simulink model "synchro_v2"  (R2020b)
settings: Solver=FixedStepAuto  StartTime=0.0  StopTime=2  FixedStep=Ts  RelTol=1e-3
values from neighbouring files (symbols this model uses):
  m = 5/100    (= 0.05)    [synchro_parameters_v1.m]
  Sbase = 1    [synchro_parameters_v1.m]
  Ts = 1/Fs    (= 0.0001)    [synchro_parameters_v1.m]
  Vbase = 1    [synchro_parameters_v1.m]
  w_droop = 10*2*pi    (= 62.8318530718)    [synchro_parameters_v1.m]
  w_pll = 10*2*pi    (= 62.8318530718)    [synchro_parameters_v1.m]
  w_tau = 1e3*2*pi    (= 6283.18530718)    [synchro_parameters_v1.m]
  Wbase = 2*pi*50    (= 314.159265359)    [synchro_parameters_v1.m]
undefined symbols (not defined in the file or in its folder): DiscIntNeverNeededParam
libraries: powerlib x36, SimplexPS x34, Simplex_PowerSystems x4
(part 1 of 2)
settings Model: Creator=admin_user  LastModifiedBy=admin_user

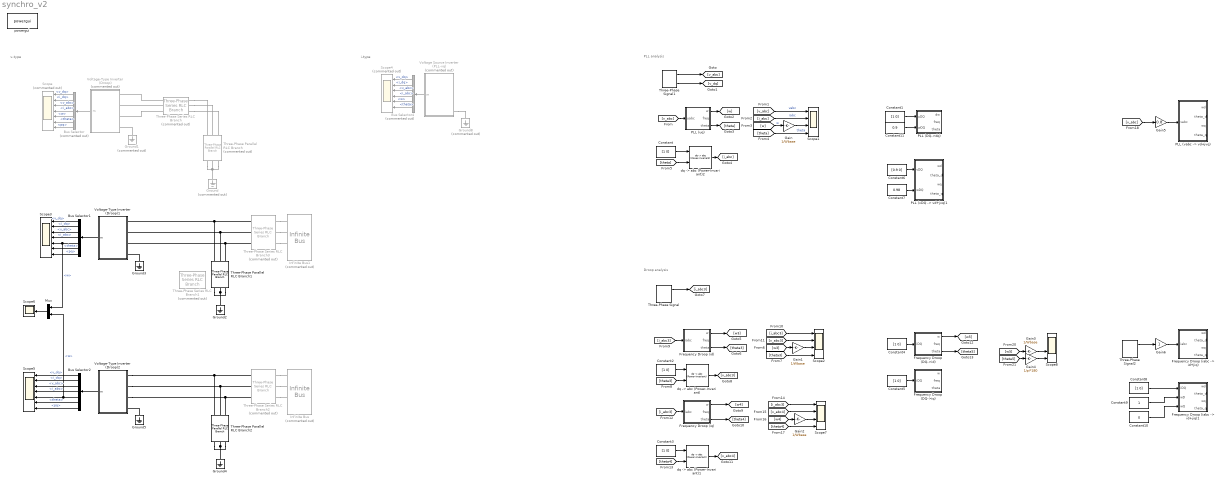
== system synchro_v2 ==
  note: Droop analysis
  note: PLL analysis
  note: i-type
  note: v-type
  Bus Selector : BusSelector  Commented=on  OutputSignals=v_dq,i_dq,v_abc,i_abc,w,theta,pq
  Bus Selector1 : BusSelector  OutputSignals=v_dq,i_dq,v_abc,i_abc,w,theta,pq
  Bus Selector2 : BusSelector  OutputSignals=v_dq,i_dq,v_abc,i_abc,w,theta,pq
  Bus Selector4 : BusSelector  Commented=on  OutputSignals=v_dq,i_dq,v_abc,i_abc,w,theta
  Constant{,1..5,8} (7 alike) : Constant  Value=[1 0]
  Constant10 : Constant  Value=0
  Constant11 : Constant  Value=0.9
  Constant6 : Constant  Value=[0.9 0]
  Constant7 : Constant  Value=0.98
  Constant9 : Constant
  "Frequency Droop (iabc -> id+jiq)" : Subsystem  AncestorBlock=|  mask{Ts=Ts, Sbase=Sbase, Vbase=Vbase, Wbase=Wbase, m=m, w_tau=w_droop, theta_d0=0, theta_q0=0, id0=0, iq0=0, wd0=1, wq0=0}
      | SimplexPS/Frequency Droop
      | (iabc -> id+jiq)
      mask prompts: Ts "Ts (s), sampling period"; Sbase "Sbase (VA), base power"; Vbase "Vbase (V), base voltage"; Wbase "Wbase (s), base frequency"; m "m (pu), droop gain"; w_tau "w_tau (pu), low-pass filter bandwidth"; theta_d0 "theta_d0 (rad/s), initial d-axis angle"; theta_q0 "theta_q0 (rad/s), initial q-axis angle"; id0 "id0 (pu), d-axis current setting point"; iq0 "iq0 (pu), q-axis current setting point"; wd0 "wd0 (pu), d-axis angular frequency setting point"; wq0 "wq0 (pu), q-axis angular frequency setting point"
  "Frequency Droop (iabc -> id+jiq)1" : Subsystem  AncestorBlock=|  mask{Ts=Ts, Sbase=Sbase, Vbase=Vbase, Wbase=Wbase, m=m, w_tau=w_droop, theta_d0=0, theta_q0=0, id0=0, iq0=0, wd0=1, wq0=0}
      | SimplexPS/Frequency Droop
      | (iabc -> id+jiq)1
      mask prompts: Ts "Ts (s), sampling period"; Sbase "Sbase (VA), base power"; Vbase "Vbase (V), base voltage"; Wbase "Wbase (s), base frequency"; m "m (pu), droop gain"; w_tau "w_tau (pu), low-pass filter bandwidth"; theta_d0 "theta_d0 (rad/s), initial d-axis angle"; theta_q0 "theta_q0 (rad/s), initial q-axis angle"; id0 "id0 (pu), d-axis current setting point"; iq0 "iq0 (pu), q-axis current setting point"; wd0 "wd0 (pu), d-axis angular frequency setting point"; wq0 "wq0 (pu), q-axis angular frequency setting point"
  Frequency Droop (DQ->id) : Subsystem  AncestorBlock=SimplexPS/Frequency Droop (id)  mask{Ts=Ts, Sbase=Sbase, Vbase=Vbase, Wbase=Wbase, m=m, w_tau=w_droop, theta0=0, P0=0, W0=1}
      mask prompts: Ts "Ts (s), samping period"; Sbase "Sbase (VA), base power"; Vbase "Vbase (V), base voltage"; Wbase "Wbase (rad/s), base angular frequency"; m "m (pu), droop gain"; w_tau "w_tau (rad/s), low-pass filter bandwidth"; theta0 "theta0 (rad), initial angle"; P0 "P0 (pu), power setting point"; W0 "W0 (pu), frequency setting point"
  Frequency Droop (DQ->iq) : Subsystem  AncestorBlock=SimplexPS/Frequency Droop (id)  mask{Ts=Ts, Sbase=Sbase, Vbase=Vbase, Wbase=Wbase, m=m, w_tau=w_droop, theta0=0, P0=0, W0=1}
      mask prompts: Ts "Ts (s), samping period"; Sbase "Sbase (VA), base power"; Vbase "Vbase (V), base voltage"; Wbase "Wbase (rad/s), base angular frequency"; m "m (pu), droop gain"; w_tau "w_tau (rad/s), low-pass filter bandwidth"; theta0 "theta0 (rad), initial angle"; P0 "P0 (pu), power setting point"; W0 "W0 (pu), frequency setting point"
  Frequency Droop (id) : Subsystem  AncestorBlock=SimplexPS/Frequency Droop (id)  mask{Ts=Ts, Sbase=Sbase, Vbase=Vbase, Wbase=Wbase, m=m, w_tau=w_droop, theta0=0, P0=0, W0=1}
      mask prompts: Ts "Ts (s), samping period"; Sbase "Sbase (VA), base power"; Vbase "Vbase (V), base voltage"; Wbase "Wbase (rad/s), base angular frequency"; m "m (pu), droop gain"; w_tau "w_tau (rad/s), low-pass filter bandwidth"; theta0 "theta0 (rad), initial angle"; P0 "P0 (pu), power setting point"; W0 "W0 (pu), frequency setting point"
  Frequency Droop (iq) : Subsystem  AncestorBlock=SimplexPS/Frequency Droop (iq)  mask{Ts=Ts, Sbase=Sbase, Vbase=Vbase, Wbase=Wbase, m=m, w_tau=w_droop, theta0=0, P0=0, W0=1}
      mask prompts: Ts "Ts (s), samping period"; Sbase "Sbase (VA), base power"; Vbase "Vbase (V), base voltage"; Wbase "Wbase (rad/s), base angular frequency"; m "m (pu), droop gain"; w_tau "w_tau (rad/s), low-pass filter bandwidth"; theta0 "theta0 (rad), initial angle"; P0 "P0 (pu), power setting point"; W0 "W0 (pu), frequency setting point"
  Gain{,1..3} (4 alike) : Gain  Gain=1/Wbase
  Gain4 : Gain  Gain=1/pi*180
  Gain5 : Gain  Gain=0.8
  Gain6 : Gain
  Ground : powerlib/Elements/Ground  Commented=on  LConnTagsString=a
  Ground1 : powerlib/Elements/Ground  Commented=on  LConnTagsString=a
  Ground{2..5} (4 alike) : powerlib/Elements/Ground  LConnTagsString=a
  Ground8 : powerlib/Elements/Ground  Commented=on  LConnTagsString=a
  Infinite Bus : SimplexPS/Infinite Bus  Commented=on  Ts=Ts  Sbase=Sbase  Vbase=Vbase  Wbase=Wbase  vd=1  vq=0  theta0=0  w=Wbase  R=1e-30
      settings: SourceProductName=Simplex Power Systems
  Infinite Bus1 : SimplexPS/Infinite Bus  Commented=on  Ts=Ts  Sbase=Sbase  Vbase=Vbase  Wbase=Wbase  vd=1  vq=0  theta0=0  w=Wbase  R=1e-30
      settings: SourceProductName=Simplex Power Systems
  Mux : Mux  Inputs=2
  "PLL (vDQ -> vd+jvq)1" : Subsystem  AncestorBlock=|  mask{Ts=Ts, Wbase=Wbase, Vbase=Vbase, w_pll=w_pll, w_tau=w_tau, theta_d0=pi/4, theta_q0=0}
      | SimplexPS/PLL
      | (vabc -> vd+jvq)
      mask prompts: Ts "Ts (s), sampling period"; Wbase "Wbase (rad/s), frequency base"; Vbase "Vbase (rad/s), voltage base"; w_pll "w_pll (rad/s), PLL bandwidth"; w_tau "w_tau (rad/s), PLL filter"; theta_d0 "theta_d0 (rad), initial d-axis angle"; theta_q0 "theta_q0 (rad), initial q-axis angle"
  "PLL (vabc -> vd+jvq)" : Subsystem  AncestorBlock=|  mask{Ts=Ts, Wbase=Wbase, Vbase=Vbase, w_pll=w_pll, w_tau=w_tau, theta_d0=pi/4, theta_q0=0}
      | SimplexPS/PLL
      | (vabc -> vd+jvq)
      mask prompts: Ts "Ts (s), sampling period"; Wbase "Wbase (rad/s), frequency base"; Vbase "Vbase (rad/s), voltage base"; w_pll "w_pll (rad/s), PLL bandwidth"; w_tau "w_tau (rad/s), PLL filter"; theta_d0 "theta_d0 (rad), initial d-axis angle"; theta_q0 "theta_q0 (rad), initial q-axis angle"
  PLL (DQ->dq) : Subsystem  AncestorBlock=SimplexPS/PLL (uq)  mask{Ts=Ts, Ubase=Vbase, Wbase=Wbase, w_pll=w_pll, w_tau=w_tau, theta0=0}
      mask prompts: Ts "Ts (s), sampling period"; Ubase "Ubase, input base, e.g., Vbase (V), Ibase (A), etc"; Wbase "Wbase (rad/s), frequency base"; w_pll "w_pll (rad/s), PLL bandwidth"; w_tau "w_tau (rad/s), low-pass filter bandwidth"; theta0 "theta0 (rad), initial angle"
  PLL (uq) : Subsystem  AncestorBlock=SimplexPS/PLL (uq)  mask{Ts=Ts, Ubase=Vbase, Wbase=Wbase, w_pll=w_pll, w_tau=w_tau, theta0=0}
      mask prompts: Ts "Ts (s), sampling period"; Ubase "Ubase, input base, e.g., Vbase (V), Ibase (A), etc"; Wbase "Wbase (rad/s), frequency base"; w_pll "w_pll (rad/s), PLL bandwidth"; w_tau "w_tau (rad/s), low-pass filter bandwidth"; theta0 "theta0 (rad), initial angle"
  Scope : Scope  Commented=on  NumInputPorts=7
  Scope{1..2,7..8} (4 alike) : Scope  NumInputPorts=4
  Scope3 : Scope  NumInputPorts=7
  Scope4 : Scope  Commented=on  NumInputPorts=6
  Scope5 : Scope  NumInputPorts=7
  Scope6 : Scope
  Three-Phase Parallel RLC Branch : powerlib/Elements/Three-Phase Parallel RLC Branch  Commented=on  LConnTagsString=A|B|C  RConnTagsString=A|B|C  BranchType=R  Resistance=1  Inductance=1e-3  Capacitance=1e-6  Measurements=None
      settings: SourceProductBaseCode=PS
  Three-Phase Parallel RLC Branch1 : powerlib/Elements/Three-Phase Parallel RLC Branch  LConnTagsString=A|B|C  RConnTagsString=A|B|C  BranchType=R  Resistance=1  Inductance=1e-3  Capacitance=1e-6  Measurements=None
      settings: SourceProductBaseCode=PS
  Three-Phase Parallel RLC Branch2 : powerlib/Elements/Three-Phase Parallel RLC Branch  LConnTagsString=A|B|C  RConnTagsString=A|B|C  BranchType=R  Resistance=1  Inductance=1e-3  Capacitance=1e-6  Measurements=None
      settings: SourceProductBaseCode=PS
  Three-Phase Series RLC Branch{,1..3} (4 alike) : powerlib/Elements/Three-Phase Series RLC Branch  Commented=on  LConnTagsString=A|B|C  RConnTagsString=A|B|C  BranchType=RL  Resistance=0.01  Inductance=0.2/(2*pi*50)  Capacitance=1e-6  Measurements=None
  Three-Phase Signal : SimplexPS/Three-Phase Signal  ud=1  uq=0  w=Wbase*1  theta0=0
      settings: SourceProductName=Simplex Power Systems
  Three-Phase Signal1 : SimplexPS/Three-Phase Signal  ud=1  uq=0  w=Wbase*0.95  theta0=0
      settings: SourceProductName=Simplex Power Systems
  Three-Phase Signal2 : SimplexPS/Three-Phase Signal  ud=1  uq=0  w=Wbase*0.98  theta0=0
      settings: SourceProductName=Simplex Power Systems
  Voltage Source Inverter (PLL-vq) : Subsystem  Commented=on  mask{Sbase=Sbase, Vbase=Vbase, Wbase=Wbase, Ts=Ts, i_d_r=1, i_q_r=0, w_pll=w_pll, w_tau=w_tau}
      mask prompts: Sbase "Sbase (VA), power base"; Vbase "Vbase (V), voltage base"; Wbase "Wbase (rad/s), frequency base"; Ts "Ts (s), samping period"; i_d_r "i_d_r (pu), d-axis current reference"; i_q_r "i_q_r (pu), q-axis current reference"; w_pll "w_pll (rad/s), PLL bandwidth"; w_tau "w_tau (rad/s), PLL filter"
  Voltage-Type Inverter (Droop) : Subsystem  Commented=on  mask{Sbase=Sbase, Vbase=Vbase, Wbase=Wbase, Ts=Ts, v_d0=1, v_q0=0, w0=1, m=m, n=0, P0=0, Q0=0, w_droop=w_droop}
      mask prompts: Sbase "Sbase (VA)"; Vbase "Vbase (V)"; Wbase "Wbase (rad/s)"; Ts "Ts (s)"; v_d0 "v_d0 (pu), d-axis voltage setting point"; v_q0 "v_q0 (pu), q-axis voltage setting point"; w0 "w0 (pu), frequency setting point"; m "m (pu), frequency droop gain"; n "n (pu), voltage droop gain"; P0 "P0 (pu), active power setting point"; Q0 "Q0 (pu), reactive power setting point"; w_droop "w_droop (rad/s), droop bandwidth"
  Voltage-Type Inverter (Droop)1 : Subsystem  mask{Sbase=Sbase, Vbase=Vbase, Wbase=Wbase, Ts=Ts, v_d0=1, v_q0=0, w0=1, m=m, n=0, P0=0, Q0=0, w_droop=w_droop}
      mask prompts: Sbase "Sbase (VA)"; Vbase "Vbase (V)"; Wbase "Wbase (rad/s)"; Ts "Ts (s)"; v_d0 "v_d0 (pu), d-axis voltage setting point"; v_q0 "v_q0 (pu), q-axis voltage setting point"; w0 "w0 (pu), frequency setting point"; m "m (pu), frequency droop gain"; n "n (pu), voltage droop gain"; P0 "P0 (pu), active power setting point"; Q0 "Q0 (pu), reactive power setting point"; w_droop "w_droop (rad/s), droop bandwidth"
  Voltage-Type Inverter (Droop)2 : Subsystem  mask{Sbase=Sbase, Vbase=Vbase, Wbase=Wbase, Ts=Ts, v_d0=1, v_q0=0, w0=1, m=m, n=0, P0=0, Q0=0, w_droop=w_droop}
      mask prompts: Sbase "Sbase (VA)"; Vbase "Vbase (V)"; Wbase "Wbase (rad/s)"; Ts "Ts (s)"; v_d0 "v_d0 (pu), d-axis voltage setting point"; v_q0 "v_q0 (pu), q-axis voltage setting point"; w0 "w0 (pu), frequency setting point"; m "m (pu), frequency droop gain"; n "n (pu), voltage droop gain"; P0 "P0 (pu), active power setting point"; Q0 "Q0 (pu), reactive power setting point"; w_droop "w_droop (rad/s), droop bandwidth"
  "dq -> abc (Power-Invariant)" : SimplexPS/dq -> abc (Power-Invariant)  SystemSampleTime=-1  VariantActivationTime=update diagram  Latency=0  AutoFrameSizeCalculation=off
      settings: SourceProductName=Simplex Power Systems
  "dq -> abc (Power-Invariant)1" : SimplexPS/dq -> abc (Power-Invariant)  SystemSampleTime=-1  VariantActivationTime=update diagram  Latency=0  AutoFrameSizeCalculation=off
      settings: SourceProductName=Simplex Power Systems
  "dq -> abc (Power-Invariant)2" : SimplexPS/dq -> abc (Power-Invariant)  SystemSampleTime=-1  VariantActivationTime=update diagram  Latency=0  AutoFrameSizeCalculation=off
      settings: SourceProductName=Simplex Power Systems
  powergui : powerlib/powergui  Priority=1  SimulationMode=Discrete  SampleTime=Ts  frequency=60  Iterations=50  frequencyindice=0  Pbase=100e6  ErrMax=1e-4  UnitsV=kV  UnitsW=MW  buscounter=0  FunctionMessages=off  echomessages=off  EnableUseOfTLC=off  CurrentSourceSwitches=off  DisableSnubberDevices=off  DisableRonSwitches=off  DisableVfSwitches=off  DisplayEquations=off  AutomaticDiscreteSolvers=off  SolverType=Tustin/Backward Euler (TBE)  Interpol=off  ExternalGateDelay=off  methode=off  Ts=100  x0status=blocks  SPID=on  SwTol=0  HookPort=off  NonlinearTolerance=1e-4  nMaxIteration=100  ContinueOnMaxIteration=off  RestoreLinks=warning  ResistiveCurrentMeasurement=off  Frange=[0:2:500]  Ylog=off  Xlog=on  ShowGrid=off  save=off  variable=ZData  structure=0  ZoomFFT=off  StartTime=0.0  cycles=1  DisplayStyle=1  fundamental=60  FreqAxis=off  MaxFrequency=1000  frequencyindicesteady=1  RmsSteady=1  display=off
  wires:
  Voltage-Type Inverter (Droop)/1(m) -> Bus Selector/1
  Bus Selector/1 -> Scope/1  "<v_dq>"
  Bus Selector/2 -> Scope/2  "<i_dq>"
  Bus Selector/3 -> Scope/3  "<v_abc>"
  Bus Selector/4 -> Scope/4  "<i_abc>"
  Bus Selector/5 -> Scope/5  "<w>"
  Bus Selector/6 -> Scope/6  "<theta>"
  Bus Selector/7 -> Scope/7  "<pq>"
  Bus Selector4/3 -> Scope4/3  "<v_abc>"
  Bus Selector4/4 -> Scope4/4  "<i_abc>"
  Bus Selector4/6 -> Scope4/6  "<theta>"
  Bus Selector4/1 -> Scope4/1  "<v_dq>"
  Voltage Source Inverter (PLL-vq)/1(m) -> Bus Selector4/1
  Bus Selector4/5 -> Scope4/5  "<w>"
  Bus Selector4/2 -> Scope4/2  "<i_dq>"
  [v_abc] -> PLL (uq)/1(uabc)
  [v_abc] -> Scope1/1  "vabc"
  PLL (uq)/3(theta) -> [theta]
  PLL (uq)/1(w) -> [w]
  [theta] -> Scope1/4  "theta"
  Constant/1 -> "dq -> abc (Power-Invariant)2"/1
  [theta] -> "dq -> abc (Power-Invariant)2"/2
  "dq -> abc (Power-Invariant)2"/1 -> [i_abc]
  [i_abc] -> Scope1/2  "iabc"
  Constant1/1 -> PLL (DQ->dq)/1(uDQ)
  Frequency Droop (id)/1(w) -> [w3]
  Frequency Droop (id)/3(theta) -> [theta3]
  [theta3] -> Scope2/4
  Three-Phase Signal/1 -> [i_abc3]
  [i_abc3] -> Frequency Droop (id)/1(iabc)
  Constant2/1 -> "dq -> abc (Power-Invariant)"/1
  [theta3] -> "dq -> abc (Power-Invariant)"/2
  "dq -> abc (Power-Invariant)"/1 -> [v_abc3]
  [i_abc3] -> Scope2/1
  [v_abc3] -> Scope2/2
  Three-Phase Signal1/1 -> [v_abc]
  Three-Phase Signal1/2 -> [v_dq]
  [w] -> Gain/1  "w"
  Gain/1 -> Scope1/3
  [w3] -> Gain1/1
  Gain1/1 -> Scope2/3
  Bus Selector1/5 -> Mux/1, Scope3/5  "<w>"
  Bus Selector1/3 -> Scope3/3  "<v_abc>"
  Bus Selector1/6 -> Scope3/6  "<theta>"
  Bus Selector1/7 -> Scope3/7  "<pq>"
  Bus Selector1/2 -> Scope3/2  "<i_dq>"
  Bus Selector1/4 -> Scope3/4  "<i_abc>"
  Bus Selector1/1 -> Scope3/1  "<v_dq>"
  Voltage-Type Inverter (Droop)1/1(m) -> Bus Selector1/1
  Bus Selector2/2 -> Scope5/2  "<i_dq>"
  Bus Selector2/4 -> Scope5/4  "<i_abc>"
  Bus Selector2/1 -> Scope5/1  "<v_dq>"
  Voltage-Type Inverter (Droop)2/1(m) -> Bus Selector2/1
  Bus Selector2/6 -> Scope5/6  "<theta>"
  Bus Selector2/3 -> Scope5/3  "<v_abc>"
  Bus Selector2/7 -> Scope5/7  "<pq>"
  Bus Selector2/5 -> Mux/2, Scope5/5  "<w>"
  Mux/1 -> Scope6/1
  [i_abc3] -> Frequency Droop (iq)/1(iabc)
  Frequency Droop (iq)/1(w) -> [w4]
  Frequency Droop (iq)/3(theta) -> [theta4]
  [theta4] -> "dq -> abc (Power-Invariant)1"/2
  Constant3/1 -> "dq -> abc (Power-Invariant)1"/1
  "dq -> abc (Power-Invariant)1"/1 -> [v_abc4]
  [theta4] -> Scope7/4
  [w4] -> Gain2/1
  [v_abc4] -> Scope7/2
  [i_abc3] -> Scope7/1
  Gain2/1 -> Scope7/3
  Constant4/1 -> Frequency Droop (DQ->id)/1(iDQ)
  Frequency Droop (DQ->id)/3(theta) -> [theta5]
  Frequency Droop (DQ->id)/1(w) -> [w5]
  Gain3/1 -> Scope8/3
  [w5] -> Gain3/1
  [theta5] -> Gain4/1
  Gain4/1 -> Scope8/4
  Constant5/1 -> Frequency Droop (DQ->iq)/1(iDQ)
  [v_abc] -> Gain5/1
  Gain5/1 -> "PLL (vabc -> vd+jvq)"/1(vabc)
  Gain6/1 -> "Frequency Droop (iabc -> id+jiq)"/1(iabc)
  Constant6/1 -> "PLL (vDQ -> vd+jvq)1"/1(vDQ)
  Constant7/1 -> "PLL (vDQ -> vd+jvq)1"/2(wDQ)
  Three-Phase Signal2/1 -> Gain6/1
  Constant8/1 -> "Frequency Droop (iabc -> id+jiq)1"/1(iDQ)
  Constant9/1 -> "Frequency Droop (iabc -> id+jiq)1"/2(wD)
  Constant10/1 -> "Frequency Droop (iabc -> id+jiq)1"/3(wQ)
  Constant11/1 -> PLL (DQ->dq)/2(wDQ)
  connections:
  Ground/LConn1 -- Three-Phase Parallel RLC Branch/RConn3 -- Three-Phase Parallel RLC Branch/RConn1 -- Three-Phase Parallel RLC Branch/RConn2
  Ground1/LConn1 -- Voltage-Type Inverter (Droop)/LConn4
  Three-Phase Series RLC Branch/RConn1 -- Three-Phase Parallel RLC Branch/LConn1
  Three-Phase Series RLC Branch/RConn2 -- Three-Phase Parallel RLC Branch/LConn2
  Three-Phase Series RLC Branch/RConn3 -- Three-Phase Parallel RLC Branch/LConn3
  Three-Phase Series RLC Branch/LConn1 -- Voltage-Type Inverter (Droop)/LConn1
  Three-Phase Series RLC Branch/LConn2 -- Voltage-Type Inverter (Droop)/LConn2
  Three-Phase Series RLC Branch/LConn3 -- Voltage-Type Inverter (Droop)/LConn3
  Voltage Source Inverter (PLL-vq)/LConn4 -- Ground8/LConn1
  Three-Phase Parallel RLC Branch1/RConn2 -- Ground2/LConn1 -- Three-Phase Parallel RLC Branch1/RConn3 -- Three-Phase Parallel RLC Branch1/RConn1
  Three-Phase Parallel RLC Branch1/LConn3 -- Voltage-Type Inverter (Droop)1/LConn3 -- Three-Phase Series RLC Branch3/LConn3
  Ground3/LConn1 -- Voltage-Type Inverter (Droop)1/LConn4
  Three-Phase Parallel RLC Branch1/LConn2 -- Voltage-Type Inverter (Droop)1/LConn2 -- Three-Phase Series RLC Branch3/LConn2
  Three-Phase Parallel RLC Branch1/LConn1 -- Voltage-Type Inverter (Droop)1/LConn1 -- Three-Phase Series RLC Branch3/LConn1
  Three-Phase Parallel RLC Branch2/RConn2 -- Ground4/LConn1 -- Three-Phase Parallel RLC Branch2/RConn3 -- Three-Phase Parallel RLC Branch2/RConn1
  Voltage-Type Inverter (Droop)2/LConn3 -- Three-Phase Series RLC Branch2/LConn3 -- Three-Phase Parallel RLC Branch2/LConn3
  Ground5/LConn1 -- Voltage-Type Inverter (Droop)2/LConn4
  Voltage-Type Inverter (Droop)2/LConn1 -- Three-Phase Parallel RLC Branch2/LConn1 -- Three-Phase Series RLC Branch2/LConn1
  Voltage-Type Inverter (Droop)2/LConn2 -- Three-Phase Series RLC Branch2/LConn2 -- Three-Phase Parallel RLC Branch2/LConn2
  Three-Phase Series RLC Branch2/RConn1 -- Infinite Bus/LConn1
  Three-Phase Series RLC Branch2/RConn2 -- Infinite Bus/LConn2
  Three-Phase Series RLC Branch2/RConn3 -- Infinite Bus/LConn3
  Three-Phase Series RLC Branch3/RConn1 -- Infinite Bus1/LConn1
  Three-Phase Series RLC Branch3/RConn3 -- Infinite Bus1/LConn3
  Three-Phase Series RLC Branch3/RConn2 -- Infinite Bus1/LConn2

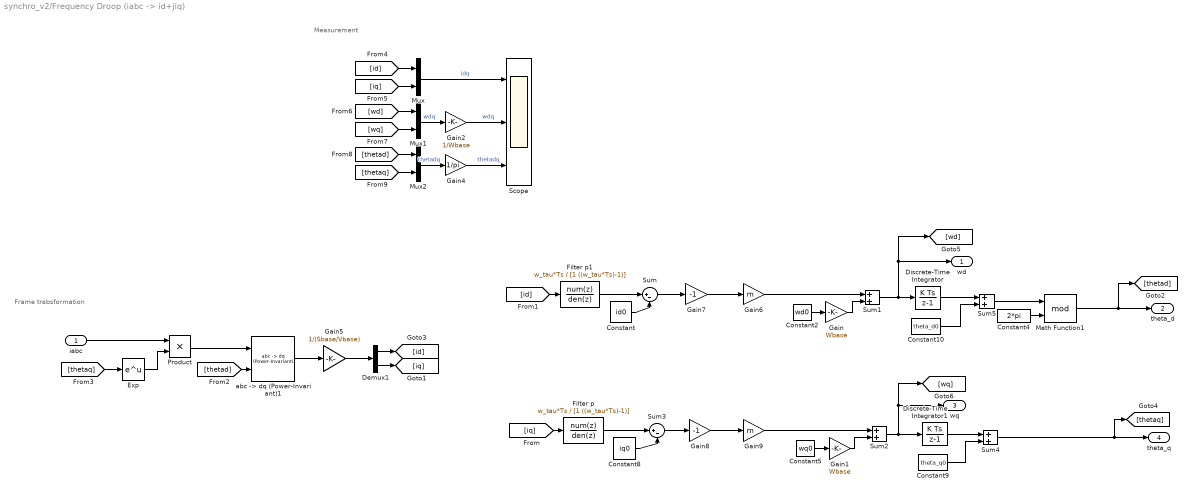
== system synchro_v2/Frequency Droop (iabc -> id+jiq) ==
  note: Frame trabsformation
  note: Measurement
  iabc : Inport
  Constant : Constant  Value=id0
  Constant10 : Constant  Value=theta_d0
  Constant2 : Constant  Value=wd0
  Constant4 : Constant  Value=2*pi
  Constant5 : Constant  Value=wq0
  Constant8 : Constant  Value=iq0
  Constant9 : Constant  Value=theta_q0
  Demux1 : Demux  Outputs=2
  Discrete-Time Integrator : DiscreteIntegrator  SampleTime=Ts  ICPrevOutput=DiscIntNeverNeededParam  ICPrevScaledInput=DiscIntNeverNeededParam
  Discrete-Time Integrator1 : DiscreteIntegrator  SampleTime=Ts  ICPrevOutput=DiscIntNeverNeededParam  ICPrevScaledInput=DiscIntNeverNeededParam
  Exp : Math  SignedPower=on  SaturateOnIntegerOverflow=on
  Filter p : DiscreteTransferFcn  Numerator=w_tau*Ts  Denominator=[1 ((w_tau*Ts)-1)]  SampleTime=Ts
  Filter p1 : DiscreteTransferFcn  Numerator=w_tau*Ts  Denominator=[1 ((w_tau*Ts)-1)]  SampleTime=Ts
  Gain : Gain  Gain=Wbase
  Gain1 : Gain  Gain=Wbase
  Gain2 : Gain  Gain=1/Wbase
  Gain4 : Gain  Gain=1/pi
  Gain5 : Gain  Gain=1/(Sbase/Vbase)
  Gain6 : Gain  Gain=m
  Gain7 : Gain  Gain=-1
  Gain8 : Gain  Gain=-1
  Gain9 : Gain  Gain=m
  Math Function1 : Math  Operator=mod  SignedPower=on  SaturateOnIntegerOverflow=on
  Mux : Mux  Inputs=2
  Mux1 : Mux  Inputs=2
  Mux2 : Mux  Inputs=2
  Product : Product
  Scope : Scope  NumInputPorts=3
  Sum : Sum  Inputs=|+-
  Sum{1..2,4..5} (4 alike) : Sum
  Sum3 : Sum  Inputs=|+-
  "abc -> dq (Power-Invariant)1" : SimplexPS/abc -> dq (Power-Invariant)  SystemSampleTime=-1  VariantActivationTime=update diagram  Latency=0  AutoFrameSizeCalculation=off
      settings: SourceProductName=Simplex Power Systems
  wd : Outport
  theta_d : Outport  Port=2
  wq : Outport  Port=3
  theta_q : Outport  Port=4
  wires:
  Gain8/1 -> Gain9/1
  Sum3/1 -> Gain8/1
  Gain7/1 -> Gain6/1
  Gain6/1 -> Sum1/1
  Gain9/1 -> Sum2/1
  Filter p1/1 -> Sum/1
  [iq] -> Filter p/1
  [wq] -> Mux1/2
  iabc/1 -> Product/1
  [id] -> Filter p1/1
  [thetad] -> "abc -> dq (Power-Invariant)1"/2
  Filter p/1 -> Sum3/1
  Discrete-Time Integrator1/1 -> Sum4/1
  Product/1 -> "abc -> dq (Power-Invariant)1"/1
  [id] -> Mux/1
  Constant10/1 -> Sum5/2
  [thetaq] -> Exp/1
  Gain/1 -> Sum1/2
  Constant5/1 -> Gain1/1
  [thetad] -> Mux2/1
  Exp/1 -> Product/2
  Mux1/1 -> Gain2/1  "wdq"
  [thetaq] -> Mux2/2
  [iq] -> Mux/2
  Constant/1 -> Sum/2
  [wd] -> Mux1/1
  Constant8/1 -> Sum3/2
  Sum5/1 -> Math Function1/1
  Demux1/1 -> [id]
  Sum4/1 -> [thetaq], theta_q/1
  Constant4/1 -> Math Function1/2
  Sum/1 -> Gain7/1
  Demux1/2 -> [iq]
  Gain4/1 -> Scope/3  "thetadq"
  Mux/1 -> Scope/1  "idq"
  Gain5/1 -> Demux1/1
  Constant9/1 -> Sum4/2
  Gain1/1 -> Sum2/2
  Mux2/1 -> Gain4/1  "thetadq"
  Sum1/1 -> Discrete-Time Integrator/1, [wd], wd/1
  Math Function1/1 -> [thetad], theta_d/1
  "abc -> dq (Power-Invariant)1"/1 -> Gain5/1
  Discrete-Time Integrator/1 -> Sum5/1
  Sum2/1 -> [wq], wq/1, Discrete-Time Integrator1/1
  Gain2/1 -> Scope/2  "wdq"
  Constant2/1 -> Gain/1

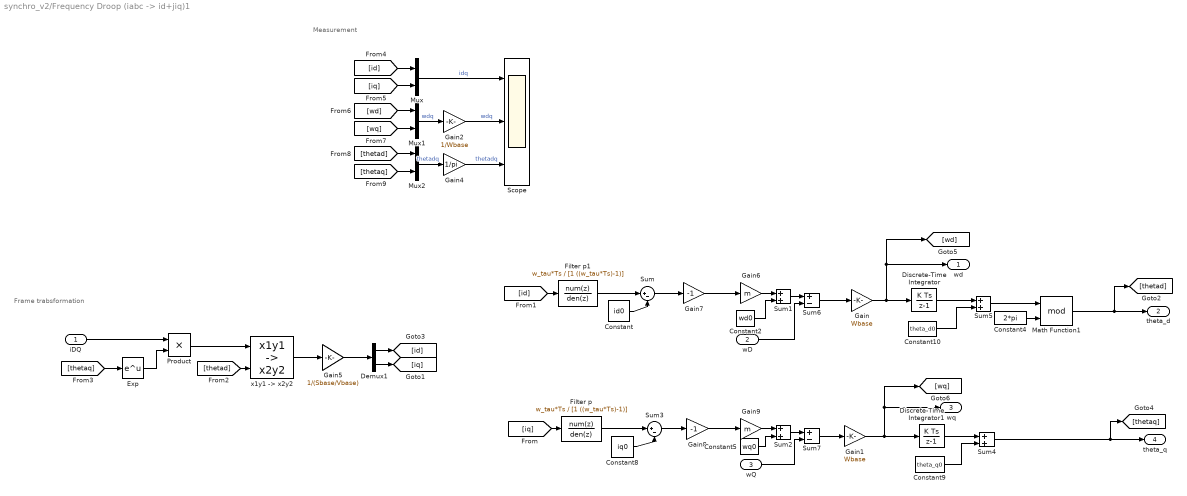
== system synchro_v2/Frequency Droop (iabc -> id+jiq)1 ==
  note: Measurement
  note: Frame trabsformation
  iDQ : Inport
  wD : Inport  Port=2
  wQ : Inport  Port=3
  Constant : Constant  Value=id0
  Constant10 : Constant  Value=theta_d0
  Constant2 : Constant  Value=wd0
  Constant4 : Constant  Value=2*pi
  Constant5 : Constant  Value=wq0
  Constant8 : Constant  Value=iq0
  Constant9 : Constant  Value=theta_q0
  Demux1 : Demux  Outputs=2
  Discrete-Time Integrator : DiscreteIntegrator  SampleTime=Ts  ICPrevOutput=DiscIntNeverNeededParam  ICPrevScaledInput=DiscIntNeverNeededParam
  Discrete-Time Integrator1 : DiscreteIntegrator  SampleTime=Ts  ICPrevOutput=DiscIntNeverNeededParam  ICPrevScaledInput=DiscIntNeverNeededParam
  Exp : Math  SignedPower=on  SaturateOnIntegerOverflow=on
  Filter p : DiscreteTransferFcn  Numerator=w_tau*Ts  Denominator=[1 ((w_tau*Ts)-1)]  SampleTime=Ts
  Filter p1 : DiscreteTransferFcn  Numerator=w_tau*Ts  Denominator=[1 ((w_tau*Ts)-1)]  SampleTime=Ts
  Gain : Gain  Gain=Wbase
  Gain1 : Gain  Gain=Wbase
  Gain2 : Gain  Gain=1/Wbase
  Gain4 : Gain  Gain=1/pi
  Gain5 : Gain  Gain=1/(Sbase/Vbase)
  Gain6 : Gain  Gain=m
  Gain7 : Gain  Gain=-1
  Gain8 : Gain  Gain=-1
  Gain9 : Gain  Gain=m
  Math Function1 : Math  Operator=mod  SignedPower=on  SaturateOnIntegerOverflow=on
  Mux : Mux  Inputs=2
  Mux1 : Mux  Inputs=2
  Mux2 : Mux  Inputs=2
  Product : Product
  Scope : Scope  NumInputPorts=3
  Sum : Sum  Inputs=|+-
  Sum{1..2,4..5} (4 alike) : Sum
  Sum3 : Sum  Inputs=|+-
  Sum6 : Sum  Inputs=+-
  Sum7 : Sum  Inputs=+-
  "x1y1 -> x2y2" : SimplexPS/x1y1 -> x2y2  SystemSampleTime=-1  VariantActivationTime=update diagram  Latency=0  AutoFrameSizeCalculation=off
      settings: SourceProductName=Simplex Power Systems
  wd : Outport
  theta_d : Outport  Port=2
  wq : Outport  Port=3
  theta_q : Outport  Port=4
  wires:
  Gain2/1 -> Scope/2  "wdq"
  Discrete-Time Integrator/1 -> Sum5/1
  "x1y1 -> x2y2"/1 -> Gain5/1
  Math Function1/1 -> theta_d/1, [thetad]
  Mux2/1 -> Gain4/1  "thetadq"
  Constant5/1 -> Sum2/2
  Constant9/1 -> Sum4/2
  Gain5/1 -> Demux1/1
  Mux/1 -> Scope/1  "idq"
  Gain4/1 -> Scope/3  "thetadq"
  Demux1/2 -> [iq]
  Sum/1 -> Gain7/1
  Constant4/1 -> Math Function1/2
  Sum4/1 -> theta_q/1, [thetaq]
  Demux1/1 -> [id]
  Sum5/1 -> Math Function1/1
  Constant8/1 -> Sum3/2
  [wd] -> Mux1/1
  Constant/1 -> Sum/2
  [iq] -> Mux/2
  [thetaq] -> Mux2/2
  Mux1/1 -> Gain2/1  "wdq"
  Exp/1 -> Product/2
  [thetad] -> Mux2/1
  Constant2/1 -> Sum1/2
  [thetaq] -> Exp/1
  Constant10/1 -> Sum5/2
  [id] -> Mux/1
  Product/1 -> "x1y1 -> x2y2"/1
  Discrete-Time Integrator1/1 -> Sum4/1
  Filter p/1 -> Sum3/1
  [thetad] -> "x1y1 -> x2y2"/2
  [id] -> Filter p1/1
  iDQ/1 -> Product/1
  [wq] -> Mux1/2
  [iq] -> Filter p/1
  Filter p1/1 -> Sum/1
  Gain9/1 -> Sum2/1
  Gain6/1 -> Sum1/1
  Gain7/1 -> Gain6/1
  Sum3/1 -> Gain8/1
  Gain8/1 -> Gain9/1
  Gain/1 -> [wd], wd/1, Discrete-Time Integrator/1
  Sum1/1 -> Sum6/1
  Sum6/1 -> Gain/1
  wD/1 -> Sum6/2
  Gain1/1 -> [wq], wq/1, Discrete-Time Integrator1/1
  Sum2/1 -> Sum7/1
  Sum7/1 -> Gain1/1
  wQ/1 -> Sum7/2

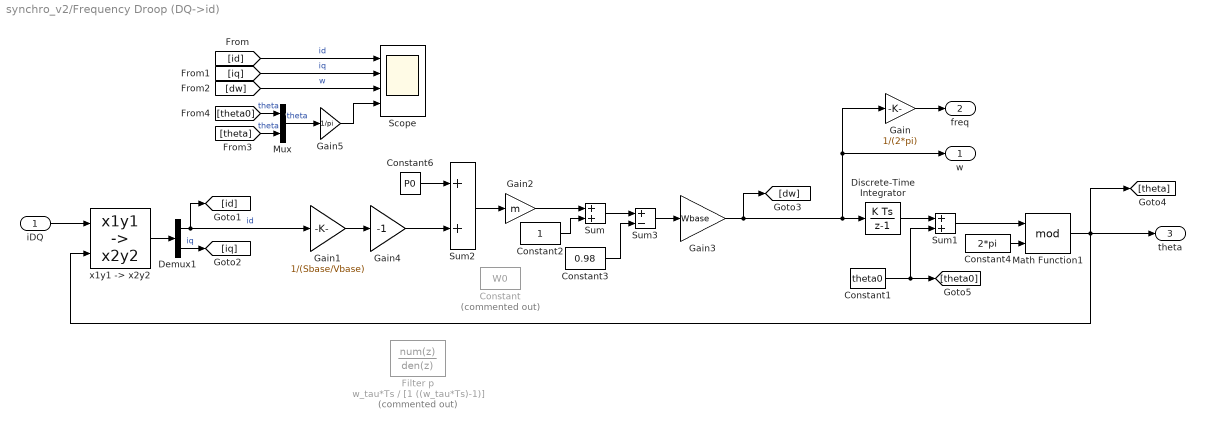
== system synchro_v2/Frequency Droop (DQ->id) ==
  iDQ : Inport
  Constant : Constant  Commented=on  Value=W0
  Constant1 : Constant  Value=theta0
  Constant2 : Constant
  Constant3 : Constant  Value=0.98
  Constant4 : Constant  Value=2*pi
  Constant6 : Constant  Value=P0
  Demux1 : Demux  Outputs=2
  Discrete-Time Integrator : DiscreteIntegrator  SampleTime=Ts  ICPrevOutput=DiscIntNeverNeededParam  ICPrevScaledInput=DiscIntNeverNeededParam
  Filter p : DiscreteTransferFcn  Commented=on  Numerator=w_tau*Ts  Denominator=[1 ((w_tau*Ts)-1)]  SampleTime=Ts
  Gain : Gain  Gain=1/(2*pi)
  Gain1 : Gain  Gain=1/(Sbase/Vbase)
  Gain2 : Gain  Gain=m
  Gain3 : Gain  Gain=Wbase
  Gain4 : Gain  Gain=-1
  Gain5 : Gain  Gain=1/pi
  Math Function1 : Math  Operator=mod  SignedPower=on  SaturateOnIntegerOverflow=on
  Mux : Mux  Inputs=2
  Scope : Scope  NumInputPorts=4
  Sum : Sum
  Sum1 : Sum
  Sum2 : Sum
  Sum3 : Sum  Inputs=+-
  "x1y1 -> x2y2" : SimplexPS/x1y1 -> x2y2  SystemSampleTime=-1  VariantActivationTime=update diagram  Latency=0  AutoFrameSizeCalculation=off
      settings: SourceProductName=Simplex Power Systems
  w : Outport
  freq : Outport  Port=2
  theta : Outport  Port=3
  wires:
  Sum1/1 -> Math Function1/1
  Math Function1/1 -> "x1y1 -> x2y2"/2, [theta], theta/1
  Gain2/1 -> Sum/1
  Discrete-Time Integrator/1 -> Sum1/1
  Gain1/1 -> Gain4/1
  "x1y1 -> x2y2"/1 -> Demux1/1
  Constant4/1 -> Math Function1/2
  iDQ/1 -> "x1y1 -> x2y2"/1
  Demux1/1 -> Gain1/1, [id]  "id"
  Constant6/1 -> Sum2/1
  Sum2/1 -> Gain2/1
  Gain/1 -> freq/1
  Gain3/1 -> [dw], w/1, Gain/1, Discrete-Time Integrator/1
  Demux1/2 -> [iq]  "iq"
  [id] -> Scope/1  "id"
  [iq] -> Scope/2  "iq"
  [dw] -> Scope/3  "w"
  Gain4/1 -> Sum2/2
  Mux/1 -> Gain5/1  "theta"
  [theta] -> Mux/2  "theta"
  [theta0] -> Mux/1  "theta"
  Constant1/1 -> [theta0], Sum1/2
  Gain5/1 -> Scope/4
  Sum/1 -> Sum3/1
  Sum3/1 -> Gain3/1
  Constant2/1 -> Sum/2
  Constant3/1 -> Sum3/2

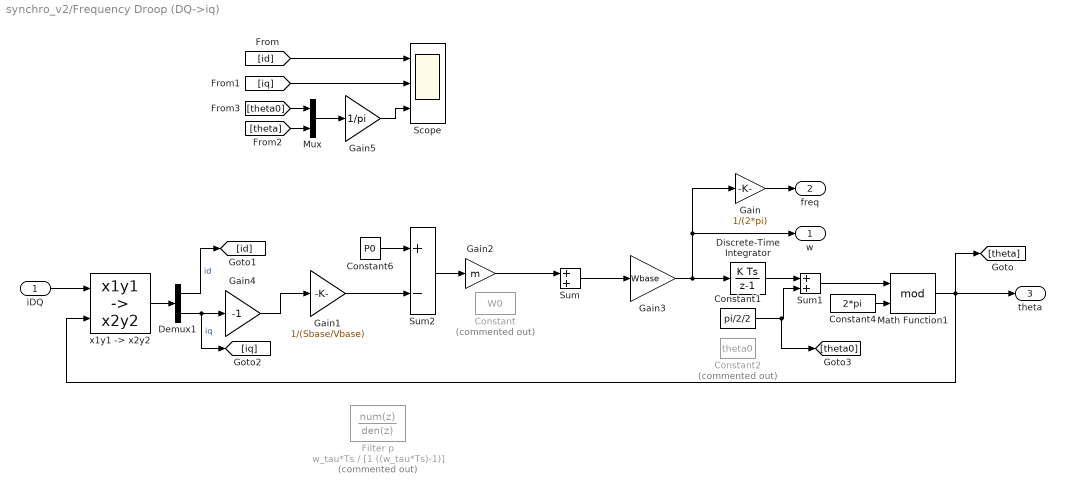
== system synchro_v2/Frequency Droop (DQ->iq) ==
  iDQ : Inport
  Constant : Constant  Commented=on  Value=W0
  Constant1 : Constant  Value=pi/2/2
  Constant2 : Constant  Commented=on  Value=theta0
  Constant4 : Constant  Value=2*pi
  Constant6 : Constant  Value=P0
  Demux1 : Demux  Outputs=2
  Discrete-Time Integrator : DiscreteIntegrator  SampleTime=Ts  ICPrevOutput=DiscIntNeverNeededParam  ICPrevScaledInput=DiscIntNeverNeededParam
  Filter p : DiscreteTransferFcn  Commented=on  Numerator=w_tau*Ts  Denominator=[1 ((w_tau*Ts)-1)]  SampleTime=Ts
  Gain : Gain  Gain=1/(2*pi)
  Gain1 : Gain  Gain=1/(Sbase/Vbase)
  Gain2 : Gain  Gain=m
  Gain3 : Gain  Gain=Wbase
  Gain4 : Gain  Gain=-1
  Gain5 : Gain  Gain=1/pi
  Math Function1 : Math  Operator=mod  SignedPower=on  SaturateOnIntegerOverflow=on
  Mux : Mux  Inputs=2
  Scope : Scope  NumInputPorts=3
  Sum : Sum
  Sum1 : Sum
  Sum2 : Sum  Inputs=+-
  "x1y1 -> x2y2" : SimplexPS/x1y1 -> x2y2  SystemSampleTime=-1  VariantActivationTime=update diagram  Latency=0  AutoFrameSizeCalculation=off
      settings: SourceProductName=Simplex Power Systems
  w : Outport
  freq : Outport  Port=2
  theta : Outport  Port=3
  wires:
  Sum1/1 -> Math Function1/1
  Math Function1/1 -> [theta], "x1y1 -> x2y2"/2, theta/1
  Gain2/1 -> Sum/1
  Discrete-Time Integrator/1 -> Sum1/1
  Gain1/1 -> Sum2/2
  "x1y1 -> x2y2"/1 -> Demux1/1
  Constant4/1 -> Math Function1/2
  iDQ/1 -> "x1y1 -> x2y2"/1
  Constant6/1 -> Sum2/1
  Sum2/1 -> Gain2/1
  Gain/1 -> freq/1
  Sum/1 -> Gain3/1
  Gain3/1 -> w/1, Gain/1, Discrete-Time Integrator/1
  Demux1/2 -> [iq], Gain4/1  "iq"
  Gain4/1 -> Gain1/1
  Constant1/1 -> [theta0], Sum1/2
  Demux1/1 -> [id]  "id"
  [id] -> Scope/1
  [theta] -> Mux/2
  [theta0] -> Mux/1
  [iq] -> Scope/2
  Mux/1 -> Gain5/1
  Gain5/1 -> Scope/3

== system synchro_v2/Frequency Droop (id) ==
  iabc : Inport
  Constant : Constant  Value=W0
  Constant2 : Constant  Value=theta0
  Constant4 : Constant  Value=2*pi
  Constant6 : Constant  Value=P0
  Demux1 : Demux  Outputs=2
  Discrete-Time Integrator : DiscreteIntegrator  SampleTime=Ts  ICPrevOutput=DiscIntNeverNeededParam  ICPrevScaledInput=DiscIntNeverNeededParam
  Filter p : DiscreteTransferFcn  Commented=on  Numerator=w_tau*Ts  Denominator=[1 ((w_tau*Ts)-1)]  SampleTime=Ts
  Gain : Gain  Gain=1/(2*pi)
  Gain1 : Gain  Gain=1/(Sbase/Vbase)
  Gain2 : Gain  Gain=m
  Gain3 : Gain  Gain=Wbase
  Gain4 : Gain  Gain=1/Wbase
  Math Function1 : Math  Operator=mod  SignedPower=on  SaturateOnIntegerOverflow=on
  Root Mean Squre : SimplexPS/Root Mean Squre  SystemSampleTime=-1  VariantActivationTime=update diagram  Latency=0  AutoFrameSizeCalculation=off
      settings: SourceProductName=Simplex Power Systems
  Scope : Scope
  Scope2 : Scope  NumInputPorts=4
  Sum : Sum
  Sum1 : Sum
  Sum2 : Sum  Inputs=+-
  "abc -> dq (Power-Invariant)" : SimplexPS/abc -> dq (Power-Invariant)  SystemSampleTime=-1  VariantActivationTime=update diagram  Latency=0  AutoFrameSizeCalculation=off
      settings: SourceProductName=Simplex Power Systems
  w : Outport
  freq : Outport  Port=2
  theta : Outport  Port=3
  wires:
  Sum1/1 -> Math Function1/1
  Constant2/1 -> Sum1/2
  Math Function1/1 -> [theta], "abc -> dq (Power-Invariant)"/2, theta/1
  Gain2/1 -> Sum/1
  Discrete-Time Integrator/1 -> Sum1/1
  Gain1/1 -> Sum2/2
  Constant/1 -> Sum/2
  "abc -> dq (Power-Invariant)"/1 -> Demux1/1
  Constant4/1 -> Math Function1/2
  iabc/1 -> "abc -> dq (Power-Invariant)"/1
  Demux1/1 -> Gain1/1, [id]  "id"
  Constant6/1 -> Sum2/1
  Sum2/1 -> Gain2/1
  Gain/1 -> freq/1
  Sum/1 -> Gain3/1
  Gain3/1 -> [w], w/1, Gain/1, Discrete-Time Integrator/1
  Demux1/2 -> [iq]
  [id] -> Root Mean Squre/1, Scope2/1  "id"
  [iq] -> Root Mean Squre/2, Scope2/2  "iq"
  [w] -> Gain4/1  "w"
  [theta] -> Scope2/4  "theta"
  Gain4/1 -> Scope2/3  "wpu"
  Root Mean Squre/1 -> Scope/1

== system synchro_v2/Frequency Droop (iq) ==
  iabc : Inport
  Constant : Constant  Value=W0
  Constant2 : Constant  Value=theta0
  Constant4 : Constant  Value=2*pi
  Constant6 : Constant  Value=P0
  Demux1 : Demux  Outputs=2
  Discrete-Time Integrator : DiscreteIntegrator  SampleTime=Ts  ICPrevOutput=DiscIntNeverNeededParam  ICPrevScaledInput=DiscIntNeverNeededParam
  Filter p : DiscreteTransferFcn  Numerator=w_tau*Ts  Denominator=[1 ((w_tau*Ts)-1)]  SampleTime=Ts
  Gain : Gain  Gain=1/(2*pi)
  Gain1 : Gain  Gain=1/(Sbase/Vbase)
  Gain2 : Gain  Gain=m
  Gain3 : Gain  Gain=Wbase
  Gain4 : Gain  Gain=-1
  Math Function1 : Math  Operator=mod  SignedPower=on  SaturateOnIntegerOverflow=on
  Scope : Scope
  Sum : Sum
  Sum1 : Sum
  Sum2 : Sum  Inputs=+-
  "abc -> dq (Power-Invariant)" : SimplexPS/abc -> dq (Power-Invariant)  SystemSampleTime=-1  VariantActivationTime=update diagram  Latency=0  AutoFrameSizeCalculation=off
      settings: SourceProductName=Simplex Power Systems
  w : Outport
  freq : Outport  Port=2
  theta : Outport  Port=3
  wires:
  Demux1/2 -> Gain4/1
  Gain3/1 -> Discrete-Time Integrator/1, Gain/1, w/1
  Sum/1 -> Gain3/1
  Gain/1 -> freq/1
  Sum2/1 -> Gain2/1
  Constant6/1 -> Sum2/1
  Gain1/1 -> Scope/1, Filter p/1
  iabc/1 -> "abc -> dq (Power-Invariant)"/1
  Constant4/1 -> Math Function1/2
  "abc -> dq (Power-Invariant)"/1 -> Demux1/1
  Constant/1 -> Sum/2
  Filter p/1 -> Sum2/2
  Discrete-Time Integrator/1 -> Sum1/1
  Gain2/1 -> Sum/1
  Math Function1/1 -> "abc -> dq (Power-Invariant)"/2, theta/1
  Constant2/1 -> Sum1/2
  Sum1/1 -> Math Function1/1
  Gain4/1 -> Gain1/1

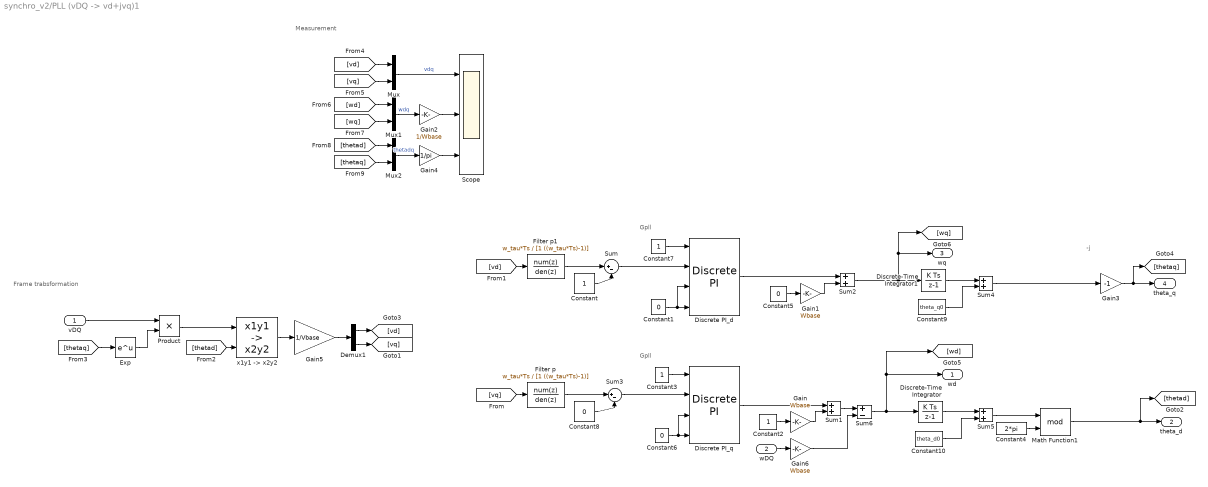
== system synchro_v2/PLL (vDQ -> vd+jvq)1 ==
  note: Measurement
  note: Frame trabsformation
  note: -j
  note: Gpll
  note: Gpll
  vDQ : Inport
  wDQ : Inport  Port=2
  Constant{,2..3,7} (4 alike) : Constant
  Constant{1,5..6,8} (4 alike) : Constant  Value=0
  Constant10 : Constant  Value=theta_d0
  Constant4 : Constant  Value=2*pi
  Constant9 : Constant  Value=theta_q0
  Demux1 : Demux  Outputs=2
  Discrete PI_d : SimplexPS/Discrete PI  Kp=w_pll  Ki=w_pll*w_pll/4  xmax=inf  xmin=-inf  Ts=Ts
      settings: SourceProductName=Simplex Power Systems
  Discrete PI_q : SimplexPS/Discrete PI  Kp=w_pll  Ki=w_pll*w_pll/4  xmax=inf  xmin=-inf  Ts=Ts
      settings: SourceProductName=Simplex Power Systems
  Discrete-Time Integrator : DiscreteIntegrator  SampleTime=Ts  ICPrevOutput=DiscIntNeverNeededParam  ICPrevScaledInput=DiscIntNeverNeededParam
  Discrete-Time Integrator1 : DiscreteIntegrator  SampleTime=Ts  ICPrevOutput=DiscIntNeverNeededParam  ICPrevScaledInput=DiscIntNeverNeededParam
  Exp : Math  SignedPower=on  SaturateOnIntegerOverflow=on
  Filter p : DiscreteTransferFcn  Numerator=w_tau*Ts  Denominator=[1 ((w_tau*Ts)-1)]  SampleTime=Ts
  Filter p1 : DiscreteTransferFcn  Numerator=w_tau*Ts  Denominator=[1 ((w_tau*Ts)-1)]  SampleTime=Ts
  Gain : Gain  Gain=Wbase
  Gain1 : Gain  Gain=Wbase
  Gain2 : Gain  Gain=1/Wbase
  Gain3 : Gain  Gain=-1
  Gain4 : Gain  Gain=1/pi
  Gain5 : Gain  Gain=1/Vbase
  Gain6 : Gain  Gain=Wbase
  Math Function1 : Math  Operator=mod  SignedPower=on  SaturateOnIntegerOverflow=on
  Mux : Mux  Inputs=2
  Mux1 : Mux  Inputs=2
  Mux2 : Mux  Inputs=2
  Product : Product
  Scope : Scope  NumInputPorts=3
  Sum : Sum  Inputs=|+-
  Sum{1..2,4..5} (4 alike) : Sum
  Sum3 : Sum  Inputs=|+-
  Sum6 : Sum  Inputs=+-
  "x1y1 -> x2y2" : SimplexPS/x1y1 -> x2y2  SystemSampleTime=-1  VariantActivationTime=update diagram  Latency=0  AutoFrameSizeCalculation=off
      settings: SourceProductName=Simplex Power Systems
  wd : Outport
  theta_d : Outport  Port=2
  wq : Outport  Port=3
  theta_q : Outport  Port=4
  wires:
  Constant4/1 -> Math Function1/2
  Constant6/1 -> Discrete PI_q/3, Discrete PI_q/4
  Demux1/2 -> [vq]
  Constant3/1 -> Discrete PI_q/1
  Math Function1/1 -> theta_d/1, [thetad]
  "x1y1 -> x2y2"/1 -> Gain5/1
  Gain5/1 -> Demux1/1
  Demux1/1 -> [vd]
  Constant/1 -> Sum/2
  Sum/1 -> Discrete PI_d/2
  Constant7/1 -> Discrete PI_d/1
  Constant1/1 -> Discrete PI_d/4, Discrete PI_d/3
  [thetad] -> "x1y1 -> x2y2"/2
  vDQ/1 -> Product/1
  Product/1 -> "x1y1 -> x2y2"/1
  Exp/1 -> Product/2
  Gain3/1 -> theta_q/1, [thetaq]
  [vq] -> Filter p/1
  [vd] -> Filter p1/1
  Filter p1/1 -> Sum/1
  [thetaq] -> Exp/1
  Discrete PI_q/1 -> Sum1/1
  Sum2/1 -> Discrete-Time Integrator1/1, wq/1, [wq]
  Discrete PI_d/1 -> Sum2/1
  Constant2/1 -> Gain/1
  Constant5/1 -> Gain1/1
  Filter p/1 -> Sum3/1
  Constant8/1 -> Sum3/2
  Sum3/1 -> Discrete PI_q/2
  Discrete-Time Integrator1/1 -> Sum4/1
  Sum4/1 -> Gain3/1
  Constant9/1 -> Sum4/2
  Gain/1 -> Sum1/2
  Gain1/1 -> Sum2/2
  Discrete-Time Integrator/1 -> Sum5/1
  Sum5/1 -> Math Function1/1
  Constant10/1 -> Sum5/2
  [vd] -> Mux/1
  [vq] -> Mux/2
  [wd] -> Mux1/1
  [wq] -> Mux1/2
  [thetad] -> Mux2/1
  [thetaq] -> Mux2/2
  Mux/1 -> Scope/1  "vdq"
  Mux1/1 -> Gain2/1  "wdq"
  Mux2/1 -> Gain4/1  "thetadq"
  Gain2/1 -> Scope/2
  Gain4/1 -> Scope/3
  Sum1/1 -> Sum6/1
  Sum6/1 -> wd/1, [wd], Discrete-Time Integrator/1
  wDQ/1 -> Gain6/1
  Gain6/1 -> Sum6/2

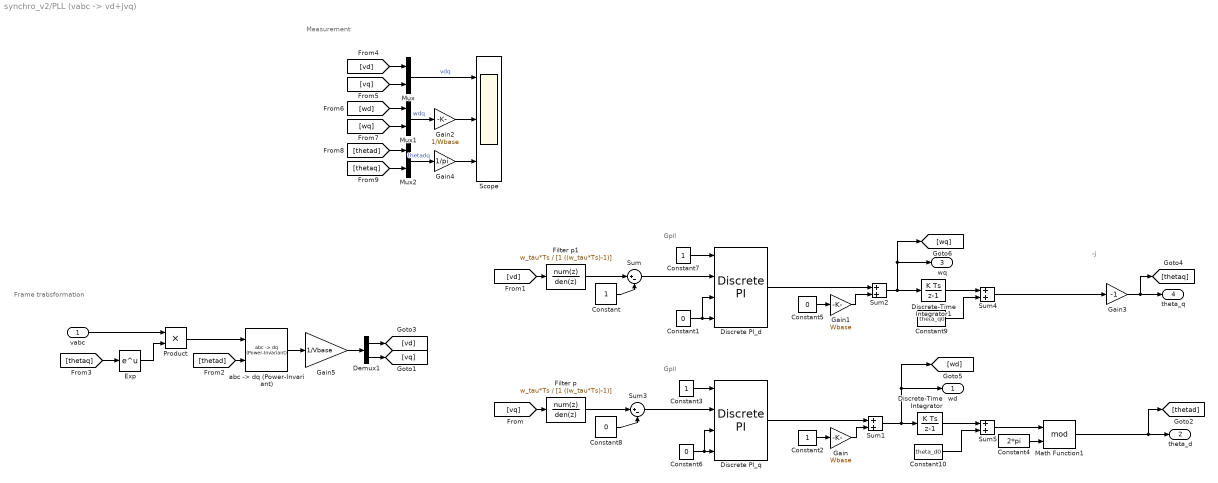
== system synchro_v2/PLL (vabc -> vd+jvq) ==
  note: Measurement
  note: Frame trabsformation
  note: -j
  note: Gpll
  note: Gpll
  vabc : Inport
  Constant{,2..3,7} (4 alike) : Constant
  Constant{1,5..6,8} (4 alike) : Constant  Value=0
  Constant10 : Constant  Value=theta_d0
  Constant4 : Constant  Value=2*pi
  Constant9 : Constant  Value=theta_q0
  Demux1 : Demux  Outputs=2
  Discrete PI_d : SimplexPS/Discrete PI  Kp=w_pll  Ki=w_pll*w_pll/4  xmax=inf  xmin=-inf  Ts=Ts
      settings: SourceProductName=Simplex Power Systems
  Discrete PI_q : SimplexPS/Discrete PI  Kp=w_pll  Ki=w_pll*w_pll/4  xmax=inf  xmin=-inf  Ts=Ts
      settings: SourceProductName=Simplex Power Systems
  Discrete-Time Integrator : DiscreteIntegrator  SampleTime=Ts  ICPrevOutput=DiscIntNeverNeededParam  ICPrevScaledInput=DiscIntNeverNeededParam
  Discrete-Time Integrator1 : DiscreteIntegrator  SampleTime=Ts  ICPrevOutput=DiscIntNeverNeededParam  ICPrevScaledInput=DiscIntNeverNeededParam
  Exp : Math  SignedPower=on  SaturateOnIntegerOverflow=on
  Filter p : DiscreteTransferFcn  Numerator=w_tau*Ts  Denominator=[1 ((w_tau*Ts)-1)]  SampleTime=Ts
  Filter p1 : DiscreteTransferFcn  Numerator=w_tau*Ts  Denominator=[1 ((w_tau*Ts)-1)]  SampleTime=Ts
  Gain : Gain  Gain=Wbase
  Gain1 : Gain  Gain=Wbase
  Gain2 : Gain  Gain=1/Wbase
  Gain3 : Gain  Gain=-1
  Gain4 : Gain  Gain=1/pi
  Gain5 : Gain  Gain=1/Vbase
  Math Function1 : Math  Operator=mod  SignedPower=on  SaturateOnIntegerOverflow=on
  Mux : Mux  Inputs=2
  Mux1 : Mux  Inputs=2
  Mux2 : Mux  Inputs=2
  Product : Product
  Scope : Scope  NumInputPorts=3
  Sum : Sum  Inputs=|+-
  Sum{1..2,4..5} (4 alike) : Sum
  Sum3 : Sum  Inputs=|+-
  "abc -> dq (Power-Invariant)" : SimplexPS/abc -> dq (Power-Invariant)  SystemSampleTime=-1  VariantActivationTime=update diagram  Latency=0  AutoFrameSizeCalculation=off
      settings: SourceProductName=Simplex Power Systems
  wd : Outport
  theta_d : Outport  Port=2
  wq : Outport  Port=3
  theta_q : Outport  Port=4
  wires:
  Constant4/1 -> Math Function1/2
  Constant6/1 -> Discrete PI_q/3, Discrete PI_q/4
  Demux1/2 -> [vq]
  Constant3/1 -> Discrete PI_q/1
  Math Function1/1 -> theta_d/1, [thetad]
  "abc -> dq (Power-Invariant)"/1 -> Gain5/1
  Gain5/1 -> Demux1/1
  Demux1/1 -> [vd]
  Constant/1 -> Sum/2
  Sum/1 -> Discrete PI_d/2
  Constant7/1 -> Discrete PI_d/1
  Constant1/1 -> Discrete PI_d/4, Discrete PI_d/3
  [thetad] -> "abc -> dq (Power-Invariant)"/2
  vabc/1 -> Product/1
  Product/1 -> "abc -> dq (Power-Invariant)"/1
  Exp/1 -> Product/2
  Gain3/1 -> theta_q/1, [thetaq]
  [vq] -> Filter p/1
  [vd] -> Filter p1/1
  Filter p1/1 -> Sum/1
  [thetaq] -> Exp/1
  Sum1/1 -> [wd], wd/1, Discrete-Time Integrator/1
  Discrete PI_q/1 -> Sum1/1
  Sum2/1 -> Discrete-Time Integrator1/1, wq/1, [wq]
  Discrete PI_d/1 -> Sum2/1
  Constant2/1 -> Gain/1
  Constant5/1 -> Gain1/1
  Filter p/1 -> Sum3/1
  Constant8/1 -> Sum3/2
  Sum3/1 -> Discrete PI_q/2
  Discrete-Time Integrator1/1 -> Sum4/1
  Sum4/1 -> Gain3/1
  Constant9/1 -> Sum4/2
  Gain/1 -> Sum1/2
  Gain1/1 -> Sum2/2
  Discrete-Time Integrator/1 -> Sum5/1
  Sum5/1 -> Math Function1/1
  Constant10/1 -> Sum5/2
  [vd] -> Mux/1
  [vq] -> Mux/2
  [wd] -> Mux1/1
  [wq] -> Mux1/2
  [thetad] -> Mux2/1
  [thetaq] -> Mux2/2
  Mux/1 -> Scope/1  "vdq"
  Mux1/1 -> Gain2/1  "wdq"
  Mux2/1 -> Gain4/1  "thetadq"
  Gain2/1 -> Scope/2
  Gain4/1 -> Scope/3

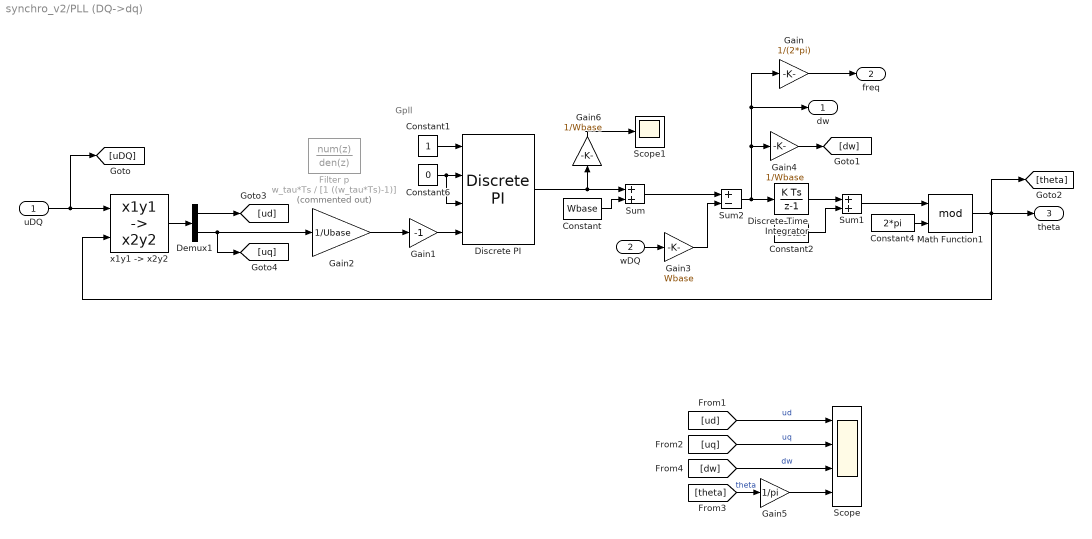
== system synchro_v2/PLL (DQ->dq) ==
  note: Gpll
  uDQ : Inport
  wDQ : Inport  Port=2
  Constant : Constant  Value=Wbase
  Constant1 : Constant
  Constant2 : Constant  Value=theta0
  Constant4 : Constant  Value=2*pi
  Constant6 : Constant  Value=0
  Demux1 : Demux  Outputs=2
  Discrete PI : SimplexPS/Discrete PI  Kp=w_pll  Ki=w_pll*w_pll/2  xmax=inf  xmin=-inf  Ts=Ts
      settings: SourceProductName=Simplex Power Systems
  Discrete-Time Integrator : DiscreteIntegrator  SampleTime=Ts  ICPrevOutput=DiscIntNeverNeededParam  ICPrevScaledInput=DiscIntNeverNeededParam
  Filter p : DiscreteTransferFcn  Commented=on  Numerator=w_tau*Ts  Denominator=[1 ((w_tau*Ts)-1)]  SampleTime=Ts
  Gain : Gain  Gain=1/(2*pi)
  Gain1 : Gain  Gain=-1
  Gain2 : Gain  Gain=1/Ubase
  Gain3 : Gain  Gain=Wbase
  Gain4 : Gain  Gain=1/Wbase
  Gain5 : Gain  Gain=1/pi
  Gain6 : Gain  Gain=1/Wbase
  Math Function1 : Math  Operator=mod  SignedPower=on  SaturateOnIntegerOverflow=on
  Scope : Scope  NumInputPorts=4
  Scope1 : Scope
  Sum : Sum
  Sum1 : Sum
  Sum2 : Sum  Inputs=+-
  "x1y1 -> x2y2" : SimplexPS/x1y1 -> x2y2  SystemSampleTime=-1  VariantActivationTime=update diagram  Latency=0  AutoFrameSizeCalculation=off
      settings: SourceProductName=Simplex Power Systems
  dw : Outport
  freq : Outport  Port=2
  theta : Outport  Port=3
  wires:
  Sum1/1 -> Math Function1/1
  Discrete-Time Integrator/1 -> Sum1/1
  Discrete PI/1 -> Gain6/1, Sum/1
  Gain1/1 -> Discrete PI/4
  Constant1/1 -> Discrete PI/1
  Constant6/1 -> Discrete PI/2, Discrete PI/3
  Demux1/2 -> [uq], Gain2/1
  Gain/1 -> freq/1
  Constant4/1 -> Math Function1/2
  "x1y1 -> x2y2"/1 -> Demux1/1
  uDQ/1 -> [uDQ], "x1y1 -> x2y2"/1
  Math Function1/1 -> "x1y1 -> x2y2"/2, theta/1, [theta]
  Gain2/1 -> Gain1/1
  Demux1/1 -> [ud]
  Constant2/1 -> Sum1/2
  Sum/1 -> Sum2/1
  Sum2/1 -> Gain4/1, dw/1, Gain/1, Discrete-Time Integrator/1
  Constant/1 -> Sum/2
  wDQ/1 -> Gain3/1
  Gain3/1 -> Sum2/2
  [ud] -> Scope/1  "ud"
  [uq] -> Scope/2  "uq"
  [dw] -> Scope/3  "dw"
  [theta] -> Gain5/1  "theta"
  Gain4/1 -> [dw]
  Gain5/1 -> Scope/4
  Gain6/1 -> Scope1/1

== system synchro_v2/PLL (uq) ==
  note: Gpll
  uabc : Inport
  Constant : Constant  Value=Wbase
  Constant1 : Constant
  Constant2 : Constant  Value=theta0
  Constant4 : Constant  Value=2*pi
  Constant6 : Constant  Value=0
  Demux1 : Demux  Outputs=2
  Discrete PI : SimplexPS/Discrete PI  Kp=w_pll  Ki=w_pll*w_pll/2  xmax=inf  xmin=-inf  Ts=Ts
      settings: SourceProductName=Simplex Power Systems
  Discrete-Time Integrator : DiscreteIntegrator  SampleTime=Ts  ICPrevOutput=DiscIntNeverNeededParam  ICPrevScaledInput=DiscIntNeverNeededParam
  Filter p : DiscreteTransferFcn  Commented=on  Numerator=w_tau*Ts  Denominator=[1 ((w_tau*Ts)-1)]  SampleTime=Ts
  Gain : Gain  Gain=1/(2*pi)
  Gain1 : Gain  Gain=-1
  Gain2 : Gain  Gain=1/Ubase
  Math Function1 : Math  Operator=mod  SignedPower=on  SaturateOnIntegerOverflow=on
  Sum : Sum
  Sum1 : Sum
  "abc -> dq (Power-Invariant)" : SimplexPS/abc -> dq (Power-Invariant)  SystemSampleTime=-1  VariantActivationTime=update diagram  Latency=0  AutoFrameSizeCalculation=off
      settings: SourceProductName=Simplex Power Systems
  w : Outport
  freq : Outport  Port=2
  theta : Outport  Port=3
  wires:
  Constant2/1 -> Sum1/2
  Sum1/1 -> Math Function1/1
  Discrete-Time Integrator/1 -> Sum1/1
  Constant/1 -> Sum/2
  Sum/1 -> Discrete-Time Integrator/1, Gain/1, w/1
  Discrete PI/1 -> Sum/1
  Gain1/1 -> Discrete PI/4
  Constant1/1 -> Discrete PI/1
  Constant6/1 -> Discrete PI/2, Discrete PI/3
  Demux1/2 -> Gain2/1
  Gain/1 -> freq/1
  Constant4/1 -> Math Function1/2
  "abc -> dq (Power-Invariant)"/1 -> Demux1/1
  uabc/1 -> "abc -> dq (Power-Invariant)"/1
  Math Function1/1 -> "abc -> dq (Power-Invariant)"/2, theta/1
  Gain2/1 -> Gain1/1

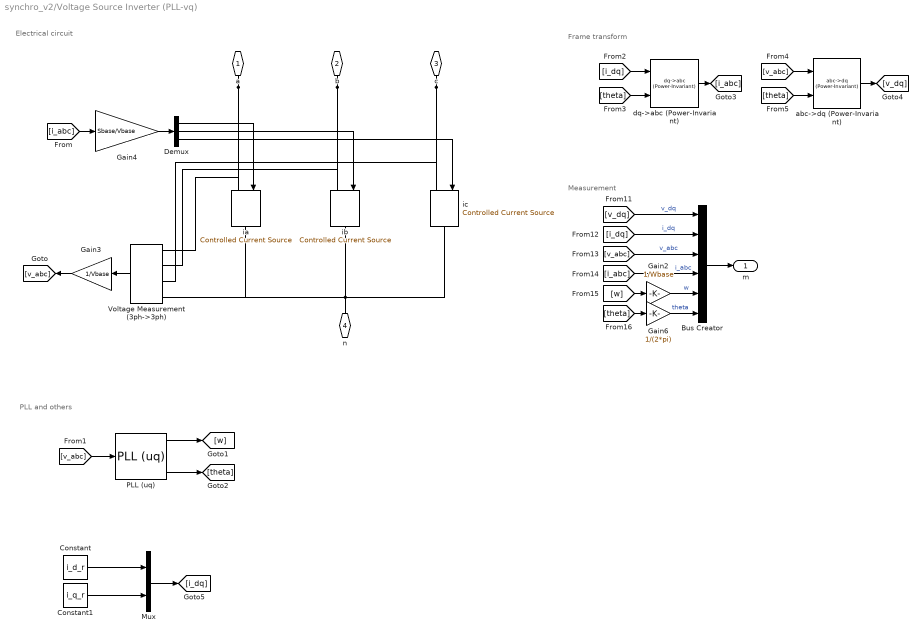
== system synchro_v2/Voltage Source Inverter (PLL-vq) ==
  note: Measurement
  note: PLL and others
  note: Frame transform
  note: Electrical circuit
  Bus Creator : BusCreator  Inputs=6
  Constant : Constant  Value=i_d_r
  Constant1 : Constant  Value=i_q_r
  Demux : Demux  Outputs=3
  Gain2 : Gain  Gain=1/Wbase
  Gain3 : Gain  Gain=1/Vbase
  Gain4 : Gain  Gain=Sbase/Vbase
  Gain6 : Gain  Gain=1/(2*pi)
  Mux : Mux  Inputs=2
  PLL (uq) : Simplex_PowerSystems/PLL (uq)  Ts=Ts  Ubase=Vbase  Wbase=Wbase  w_pll=w_pll  w_tau=w_tau  theta0=-pi/2
      settings: SourceProductName=Simplex Power Systems
  Voltage Measurement (3ph->3ph) : Simplex_PowerSystems/Voltage Measurement (3ph->3ph)  SystemSampleTime=-1  VariantActivationTime=update diagram  Latency=0  AutoFrameSizeCalculation=off
      settings: SourceProductName=Simplex Power Systems
  abc->dq (Power-Invariant) : Simplex_PowerSystems/abc->dq (Power-Invariant)  SystemSampleTime=-1  VariantActivationTime=update diagram  Latency=0  AutoFrameSizeCalculation=off
      settings: SourceProductName=Simplex Power Systems
  dq->abc (Power-Invariant) : Simplex_PowerSystems/dq->abc (Power-Invariant)  SystemSampleTime=-1  VariantActivationTime=update diagram  Latency=0  AutoFrameSizeCalculation=off
      settings: SourceProductName=Simplex Power Systems
  ia : powerlib/Electrical Sources/Controlled Current Source  Initialize=on  Source_Type=AC  Amplitude=0  Phase=0  Frequency=0  Measurements=None
  ib : powerlib/Electrical Sources/Controlled Current Source  Initialize=on  Source_Type=AC  Amplitude=0  Phase=0  Frequency=0  Measurements=None
  ic : powerlib/Electrical Sources/Controlled Current Source  Initialize=on  Source_Type=AC  Amplitude=0  Phase=0  Frequency=0  Measurements=None
  a : PMIOPort  Side=Left
  b : PMIOPort  Port=2  Side=Left
  c : PMIOPort  Port=3  Side=Left
  n : PMIOPort  Port=4  Side=Left
  m : Outport
  wires:
  [v_dq] -> Bus Creator/1  "v_dq"
  [i_dq] -> Bus Creator/2  "i_dq"
  [v_abc] -> Bus Creator/3  "v_abc"
  [i_abc] -> Bus Creator/4  "i_abc"
  Bus Creator/1 -> m/1
  [w] -> Gain2/1
  Gain2/1 -> Bus Creator/5  "w"
  [i_abc] -> Gain4/1
  Gain4/1 -> Demux/1
  [theta] -> Gain6/1
  Gain6/1 -> Bus Creator/6  "theta"
  Demux/1 -> ia/1
  Demux/2 -> ib/1
  Demux/3 -> ic/1
  Gain3/1 -> [v_abc]
  [v_abc] -> PLL (uq)/1
  PLL (uq)/1 -> [w]
  PLL (uq)/3 -> [theta]
  Voltage Measurement (3ph->3ph)/1 -> Gain3/1
  dq->abc (Power-Invariant)/1 -> [i_abc]
  [i_dq] -> dq->abc (Power-Invariant)/1
  [theta] -> dq->abc (Power-Invariant)/2
  [v_abc] -> abc->dq (Power-Invariant)/1
  [theta] -> abc->dq (Power-Invariant)/2
  abc->dq (Power-Invariant)/1 -> [v_dq]
  Constant/1 -> Mux/1
  Constant1/1 -> Mux/2
  Mux/1 -> [i_dq]
  connections:
  a/RConn1 -- ia/LConn1 -- Voltage Measurement (3ph->3ph)/LConn1
  ib/RConn1 -- ic/RConn1 -- n/RConn1 -- ia/RConn1 -- Voltage Measurement (3ph->3ph)/LConn4
  b/RConn1 -- ib/LConn1 -- Voltage Measurement (3ph->3ph)/LConn2
  c/RConn1 -- ic/LConn1 -- Voltage Measurement (3ph->3ph)/LConn3
